simulink model "control_ident_3"  (Simulink 4.00)
settings: Solver=ode45  StartTime=0.0  StopTime=10.0  RelTol=1e-3
values from neighbouring files (symbols this model uses):
  a = 1    [control_ident3.m]    (also in control_ident31.m; ident_1.m = my_sys1.den{1,:}; ident_2.m = my_sys1.den{1,:}; ident_3.m = my_sys1.den{1,:})
libraries: cstblocks x1
settings Model: LastModifiedBy=Administrator  BlockReductionOpt=off

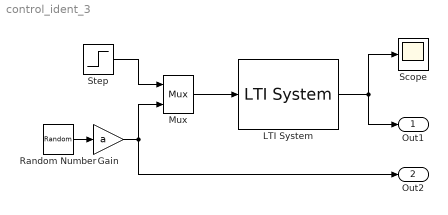
== system control_ident_3 ==
  Gain : Gain  Gain=a  Multiplication=Element-wise(K.*u)  SaturateOnIntegerOverflow=on
  LTI System : cstblocks/LTI System  sys=my_sys_lti  IC=0
  Mux : Mux  Inputs=2
      settings: DisplayOption=none
  Random Number : RandomNumber  Mean=0  Variance=1  Seed=0  SampleTime=0
  Scope : Scope
      settings: TimeRange=auto  YMin=-5  YMax=5  SaveToWorkspace=off  SaveName=ScopeData  LimitDataPoints=on  MaxDataPoints=5000
  Step : Step  Time=0  Before=0  After=1  SampleTime=0
  Out1 : Outport  Port=1
  Out2 : Outport  Port=2
  wires:
  Step/1 -> Mux/1
  Random Number/1 -> Gain/1
  Mux/1 -> LTI System/1
  LTI System/1 -> Scope/1, Out1/1
  Gain/1 -> Mux/2, Out2/1
